simulink library "Sedea_Sul_filterlib"  (R2015b)
settings: Solver=VariableStepAuto  StartTime=0.0  StopTime=10.0  RelTol=1e-3
settings Model: Creator=sedur  LastModifiedBy=sedur

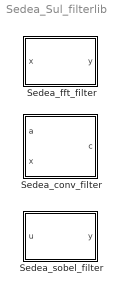
== system Sedea_Sul_filterlib ==
  Sedea_conv_filter : Subsystem  TreatAsAtomicUnit=on  mask{shape=full}
      mask TypeOptions shape: full | same | valid
      mask Display:
      | disp('myconv');
      | port_label('output', 1, 'c');
      | port_label('input', 1, 'a');
      | port_label('input', 2, 'x');
  Sedea_fft_filter : MATLAB Function  TreatAsAtomicUnit=on
  Sedea_sobel_filter : MATLAB Function  TreatAsAtomicUnit=on

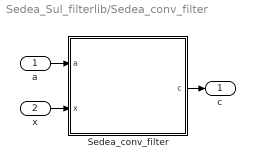
== system Sedea_Sul_filterlib/Sedea_conv_filter ==
  a : Inport
  x : Inport  Port=2
  Sedea_conv_filter : MATLAB Function  TreatAsAtomicUnit=on
  c : Outport
  wires:
  a/1 -> Sedea_conv_filter/1(a)
  x/1 -> Sedea_conv_filter/2(x)
  Sedea_conv_filter/1(c) -> c/1

== matlab function Sedea_Sul_filterlib/Sedea_sobel_filter ==
  data: u input; y output
function y = Sedea_sobel_filter(u)
%#codegen

y = sedea_sobel(u);

== matlab function Sedea_Sul_filterlib/Sedea_fft_filter ==
  data: x input; y output
function y = Sedea_fft_filter(x)
%#codegen

y = fft(x);

== matlab function Sedea_Sul_filterlib/Sedea_conv_filter/Sedea_conv_filter ==
  data: a input; c output; x input; shape parameter
function c = Sedea_conv_filter(a, x, shape)
%#codegen
if shape == 1
    c = conv(a, x, 'full');
elseif shape == 2
    c = conv(a, x, 'same');
else
    c = conv(a, x, 'valid');
end
